simulink model "Receive1"  (R2021a)
settings: Solver=VariableStepAuto  StartTime=0.0  StopTime=20000  RelTol=1e-3
values from neighbouring files (symbols this model uses):
  n_overlapped_channel = 2 * 1024    (= 2048)    [receive1_script.m]
  parallel_factor = 4    [receive1_script.m]
libraries: xbsIndex_r4 x522, xrbsSSR_Library x15, dspsrcs4 x12
(part 4 of 4)

== system Receive1/binSelect/slice_and_sel3 ==
  sel : Inport
  data_in : Inport  Port=2
  Mux2 : xbsIndex_r4/Mux  inputs=4  en=off  latency=1  precision=Full  arith_type=Unsigned  n_bits=16  bin_pt=14  quantization=Truncate  overflow=Wrap  dbl_ovrd=off  block_type=mux
  Slice QI_0 : xbsIndex_r4/Slice  nbits=27*2  boolean_output=off  mode=Lower Bit Location + Width  bit1=0  base1=MSB of Input  bit0=0  base0=LSB of Input  dbl_ovrd=off  block_type=slice
  Slice QI_1 : xbsIndex_r4/Slice  nbits=27*2  boolean_output=off  mode=Lower Bit Location + Width  bit1=0  base1=MSB of Input  bit0=27*2  base0=LSB of Input  dbl_ovrd=off  block_type=slice
  Slice QI_2 : xbsIndex_r4/Slice  nbits=27*2  boolean_output=off  mode=Lower Bit Location + Width  bit1=0  base1=MSB of Input  bit0=27*4  base0=LSB of Input  dbl_ovrd=off  block_type=slice
  Slice QI_3 : xbsIndex_r4/Slice  nbits=27*2  boolean_output=off  mode=Lower Bit Location + Width  bit1=0  base1=MSB of Input  bit0=27*6  base0=LSB of Input  dbl_ovrd=off  block_type=slice
  data_out : Outport
  wires:
  Mux2/1 -> data_out/1
  Slice QI_2/1 -> Mux2/4
  Slice QI_1/1 -> Mux2/3
  Slice QI_3/1 -> Mux2/5
  sel/1 -> Mux2/1
  Slice QI_0/1 -> Mux2/2
  data_in/1 -> Slice QI_0/1, Slice QI_1/1, Slice QI_2/1, Slice QI_3/1

== system Receive1/binSelect/slice_and_sel4 ==
  sel : Inport
  data_in : Inport  Port=2
  Mux2 : xbsIndex_r4/Mux  inputs=4  en=off  latency=1  precision=Full  arith_type=Unsigned  n_bits=16  bin_pt=14  quantization=Truncate  overflow=Wrap  dbl_ovrd=off  block_type=mux
  Slice QI_0 : xbsIndex_r4/Slice  nbits=27*2  boolean_output=off  mode=Lower Bit Location + Width  bit1=0  base1=MSB of Input  bit0=0  base0=LSB of Input  dbl_ovrd=off  block_type=slice
  Slice QI_1 : xbsIndex_r4/Slice  nbits=27*2  boolean_output=off  mode=Lower Bit Location + Width  bit1=0  base1=MSB of Input  bit0=27*2  base0=LSB of Input  dbl_ovrd=off  block_type=slice
  Slice QI_2 : xbsIndex_r4/Slice  nbits=27*2  boolean_output=off  mode=Lower Bit Location + Width  bit1=0  base1=MSB of Input  bit0=27*4  base0=LSB of Input  dbl_ovrd=off  block_type=slice
  Slice QI_3 : xbsIndex_r4/Slice  nbits=27*2  boolean_output=off  mode=Lower Bit Location + Width  bit1=0  base1=MSB of Input  bit0=27*6  base0=LSB of Input  dbl_ovrd=off  block_type=slice
  data_out : Outport
  wires:
  data_in/1 -> Slice QI_3/1, Slice QI_2/1, Slice QI_1/1, Slice QI_0/1
  Slice QI_0/1 -> Mux2/2
  sel/1 -> Mux2/1
  Slice QI_3/1 -> Mux2/5
  Slice QI_1/1 -> Mux2/3
  Slice QI_2/1 -> Mux2/4
  Mux2/1 -> data_out/1

== system Receive1/binSelect/slice_and_sel5 ==
  sel : Inport
  data_in : Inport  Port=2
  Mux2 : xbsIndex_r4/Mux  inputs=4  en=off  latency=1  precision=Full  arith_type=Unsigned  n_bits=16  bin_pt=14  quantization=Truncate  overflow=Wrap  dbl_ovrd=off  block_type=mux
  Slice QI_0 : xbsIndex_r4/Slice  nbits=27*2  boolean_output=off  mode=Lower Bit Location + Width  bit1=0  base1=MSB of Input  bit0=0  base0=LSB of Input  dbl_ovrd=off  block_type=slice
  Slice QI_1 : xbsIndex_r4/Slice  nbits=27*2  boolean_output=off  mode=Lower Bit Location + Width  bit1=0  base1=MSB of Input  bit0=27*2  base0=LSB of Input  dbl_ovrd=off  block_type=slice
  Slice QI_2 : xbsIndex_r4/Slice  nbits=27*2  boolean_output=off  mode=Lower Bit Location + Width  bit1=0  base1=MSB of Input  bit0=27*4  base0=LSB of Input  dbl_ovrd=off  block_type=slice
  Slice QI_3 : xbsIndex_r4/Slice  nbits=27*2  boolean_output=off  mode=Lower Bit Location + Width  bit1=0  base1=MSB of Input  bit0=27*6  base0=LSB of Input  dbl_ovrd=off  block_type=slice
  data_out : Outport
  wires:
  Mux2/1 -> data_out/1
  Slice QI_2/1 -> Mux2/4
  Slice QI_1/1 -> Mux2/3
  Slice QI_3/1 -> Mux2/5
  sel/1 -> Mux2/1
  Slice QI_0/1 -> Mux2/2
  data_in/1 -> Slice QI_0/1, Slice QI_1/1, Slice QI_2/1, Slice QI_3/1

== system Receive1/binSelect/slice_and_sel6 ==
  sel : Inport
  data_in : Inport  Port=2
  Mux2 : xbsIndex_r4/Mux  inputs=4  en=off  latency=1  precision=Full  arith_type=Unsigned  n_bits=16  bin_pt=14  quantization=Truncate  overflow=Wrap  dbl_ovrd=off  block_type=mux
  Slice QI_0 : xbsIndex_r4/Slice  nbits=27*2  boolean_output=off  mode=Lower Bit Location + Width  bit1=0  base1=MSB of Input  bit0=0  base0=LSB of Input  dbl_ovrd=off  block_type=slice
  Slice QI_1 : xbsIndex_r4/Slice  nbits=27*2  boolean_output=off  mode=Lower Bit Location + Width  bit1=0  base1=MSB of Input  bit0=27*2  base0=LSB of Input  dbl_ovrd=off  block_type=slice
  Slice QI_2 : xbsIndex_r4/Slice  nbits=27*2  boolean_output=off  mode=Lower Bit Location + Width  bit1=0  base1=MSB of Input  bit0=27*4  base0=LSB of Input  dbl_ovrd=off  block_type=slice
  Slice QI_3 : xbsIndex_r4/Slice  nbits=27*2  boolean_output=off  mode=Lower Bit Location + Width  bit1=0  base1=MSB of Input  bit0=27*6  base0=LSB of Input  dbl_ovrd=off  block_type=slice
  data_out : Outport
  wires:
  Mux2/1 -> data_out/1
  Slice QI_2/1 -> Mux2/4
  Slice QI_1/1 -> Mux2/3
  Slice QI_3/1 -> Mux2/5
  sel/1 -> Mux2/1
  Slice QI_0/1 -> Mux2/2
  data_in/1 -> Slice QI_0/1, Slice QI_1/1, Slice QI_2/1, Slice QI_3/1

== system Receive1/binSelect/slice_and_sel7 ==
  sel : Inport
  data_in : Inport  Port=2
  Mux2 : xbsIndex_r4/Mux  inputs=4  en=off  latency=1  precision=Full  arith_type=Unsigned  n_bits=16  bin_pt=14  quantization=Truncate  overflow=Wrap  dbl_ovrd=off  block_type=mux
  Slice QI_0 : xbsIndex_r4/Slice  nbits=27*2  boolean_output=off  mode=Lower Bit Location + Width  bit1=0  base1=MSB of Input  bit0=0  base0=LSB of Input  dbl_ovrd=off  block_type=slice
  Slice QI_1 : xbsIndex_r4/Slice  nbits=27*2  boolean_output=off  mode=Lower Bit Location + Width  bit1=0  base1=MSB of Input  bit0=27*2  base0=LSB of Input  dbl_ovrd=off  block_type=slice
  Slice QI_2 : xbsIndex_r4/Slice  nbits=27*2  boolean_output=off  mode=Lower Bit Location + Width  bit1=0  base1=MSB of Input  bit0=27*4  base0=LSB of Input  dbl_ovrd=off  block_type=slice
  Slice QI_3 : xbsIndex_r4/Slice  nbits=27*2  boolean_output=off  mode=Lower Bit Location + Width  bit1=0  base1=MSB of Input  bit0=27*6  base0=LSB of Input  dbl_ovrd=off  block_type=slice
  data_out : Outport
  wires:
  Mux2/1 -> data_out/1
  Slice QI_2/1 -> Mux2/4
  Slice QI_1/1 -> Mux2/3
  Slice QI_3/1 -> Mux2/5
  sel/1 -> Mux2/1
  Slice QI_0/1 -> Mux2/2
  data_in/1 -> Slice QI_0/1, Slice QI_1/1, Slice QI_2/1, Slice QI_3/1
